simulink model "MODELODETURBINADERIO2017aV2"  (R2017b)
settings: Solver=FixedStepAuto  StartTime=0.0  StopTime=500  FixedStep=50e-3  RelTol=1e-3
values from neighbouring files (symbols this model uses):
  a = 790.51    [MODELOHIDRO.m]    (also in MODELOHIDROV2.m; MODELOHIDROV3.m)
  A = pi()*((D/2)^2)    [MODELOHIDRO.m]    (also in MODELOHIDROV10.m; MODELOHIDROV2.m; MODELOHIDROV3.m; MODELOHIDROV4.m)
  B = 0    [MODELOHIDRO.m]    (also in MODELOHIDROV10.m; MODELOHIDROV2.m; MODELOHIDROV3.m; MODELOHIDROV4.m)
  b = 6900.50    (= 6900.5)    [MODELOHIDRO.m]    (also in MODELOHIDROV2.m; MODELOHIDROV3.m)
  beta = 0    [MODELOHIDRO.m]    (also in MODELOHIDROV10.m; MODELOHIDROV2.m; MODELOHIDROV3.m; MODELOHIDROV4.m)
  Bi = 0.2287    [MODELOHIDRO.m]    (also in MODELOHIDROV10.m = 0.1; MODELOHIDROV2.m; MODELOHIDROV3.m; MODELOHIDROV4.m = 0.005)
  c = 23794    [MODELOHIDRO.m]    (also in MODELOHIDROV2.m; MODELOHIDROV3.m)
  d = 39268    [MODELOHIDRO.m]    (also in MODELOHIDROV2.m; MODELOHIDROV3.m)
  den = 1000    [MODELOHIDRO.m]    (also in MODELOHIDROV10.m; MODELOHIDROV2.m; MODELOHIDROV3.m; MODELOHIDROV4.m)
  e = 31863    [MODELOHIDRO.m]    (also in MODELOHIDROV2.m; MODELOHIDROV3.m)
  f = 10049    [MODELOHIDRO.m]    (also in MODELOHIDROV2.m; MODELOHIDROV3.m)
  J = 16.1919e-4    (= 0.00161919)    [MODELOHIDROV10.m]    (also in MODELOHIDROV2.m = 100; MODELOHIDROV3.m = 10; MODELOHIDROV4.m; MODELOHIDROV7.m)
  Ji = 1    [MODELOHIDRO.m]    (also in MODELOHIDROV10.m = 1.72; MODELOHIDROV2.m; MODELOHIDROV3.m; MODELOHIDROV4.m = 0.0465)
  k = 1    [MODELOHIDRO.m]    (also in MODELOHIDROV2.m; MODELOHIDROV3.m)
  Kb = 1.8    [MODELOHIDRO.m]    (also in MODELOHIDROV10.m = 6.2; MODELOHIDROV2.m; MODELOHIDROV3.m; MODELOHIDROV4.m = 0.027)
  Kp = 0.4    [MODELOHIDRO.m]    (also in MODELOHIDROV10.m = 5.6627; MODELOHIDROV2.m; MODELOHIDROV3.m; MODELOHIDROV4.m = 0.027)
  L_d = 38e-3    (= 0.038)    [MODELOHIDROV2.m]    (also in MODELOHIDROV3.m; MODELOHIDROV4.m; MODELOHIDROV7.m)
  L_q = 9.03e-3    (= 0.00903)    [MODELOHIDROV2.m]    (also in MODELOHIDROV3.m; MODELOHIDROV4.m; MODELOHIDROV7.m)
  Lambda = 0.48    [MODELOHIDROV2.m]    (also in MODELOHIDROV3.m; MODELOHIDROV4.m; MODELOHIDROV7.m)
  m = 5    [MODELOHIDRO.m]    (also in MODELOHIDROV2.m; MODELOHIDROV3.m)
  r = D/2    (= 0.5)    [MODELOHIDRO.m]    (also in MODELOHIDROV10.m; MODELOHIDROV2.m; MODELOHIDROV3.m; MODELOHIDROV4.m)
  Ri = 0.6    [MODELOHIDRO.m]    (also in MODELOHIDROV10.m = 0.973; MODELOHIDROV2.m; MODELOHIDROV3.m; MODELOHIDROV4.m = 1)
  Rs = 1.649    [MODELOHIDROV2.m]    (also in MODELOHIDROV3.m; MODELOHIDROV4.m; MODELOHIDROV7.m)
  T_d = 0    [MODELOHIDRO.m]    (also in MODELOHIDROV10.m; MODELOHIDROV2.m; MODELOHIDROV3.m; MODELOHIDROV4.m)
  z = 2    [MODELOHIDRO.m]    (also in MODELOHIDROV2.m; MODELOHIDROV3.m)
undefined symbols (not defined in the file or in its folder): sigbuilder_block
libraries: simulink x1
settings Model: Creator=zni.uao  LastModifiedBy=Hp 14
settings CodeAppCC: StateflowObjectComments=on
settings SimscapeCC: SimscapeNormalizeSystem=off

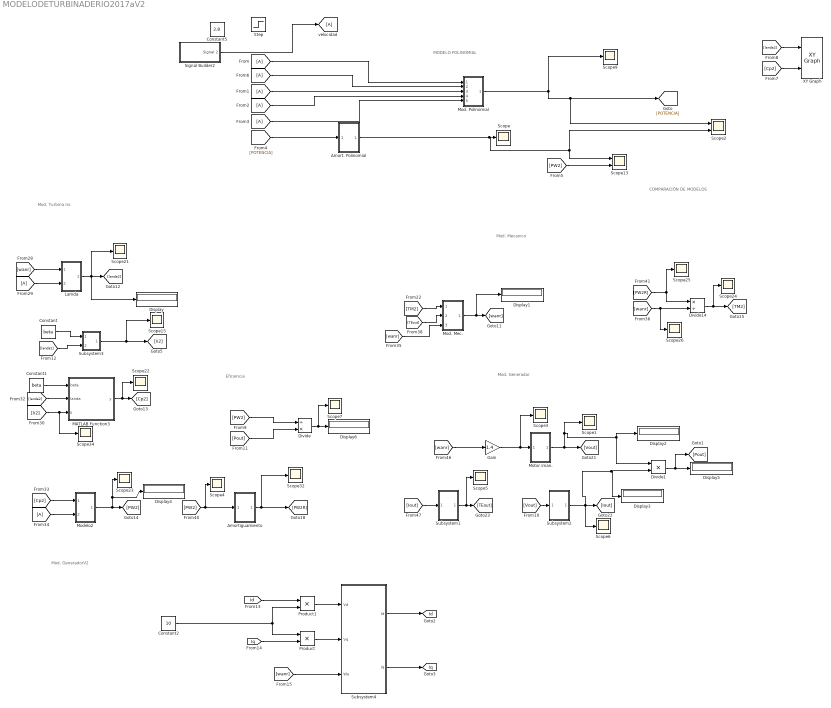
== system MODELODETURBINADERIO2017aV2 ==
  note: Mod. Generador
  note: MODELO POLINOMIAL
  note: COMPARACIÓN DE MODELOS
  note: Mod. Turbina rio
  note: Mod. Mecanico
  note: Mod. GeneradorV2
  note: Eficiencia
  Amort. Polinomial : Subsystem
  Amortiguamiento : Subsystem
  Constant : Constant  Value=beta
  Constant1 : Constant  Value=beta
  Constant2 : Constant  Value=10
  Constant5 : Constant  Value=2.8
  Display{,1..6} (7 alike) : Display
  Divide : Product  Inputs=/*
  Divide1 : Product  Inputs=**
  Divide14 : Product  Inputs=*/
  Gain : Gain  Gain=1.4
  Lamda : Subsystem
  MATLAB Function3 : MATLAB Function  TreatAsAtomicUnit=on
  Mod. Mec. : Subsystem
  Mod. Polinomial : Subsystem
  Modelo2 : Subsystem
  Motor iman. : Subsystem
  Product : Product
  Product1 : Product
  Scope{,1,3..7,9,15,21..26,32,34} (17 alike) : Scope
  Scope13 : Scope  NumInputPorts=2
  Scope2 : Scope  NumInputPorts=2
  Signal Builder2 : Subsystem  Tag=STV Subsys  LoadFcn=sigbuilder_block('load');  StartFcn=sigbuilder_block('start');  StopFcn=sigbuilder_block('stop');  ClipboardFcn=sigbuilder_block('clipboard');  mask(Sigbuilder block){tuvar=[0:10]}
      mask help: Simulink:masks:SigbuilderBlock_MD
      mask init:
      | if ~strcmp(get_param(bdroot(gcbh),'SimulationStatus'),'stopped') tuvar = sigbuilder_block('maskInit'); end
      settings: CopyFcn=sigbuilder_block('copy');  DeleteFcn=sigbuilder_block('delete');  ModelCloseFcn=sigbuilder_block('modelClose');  PreSaveFcn=sigbuilder_block('preSave');  PauseFcn=sigbuilder_block('pause');  ContinueFcn=sigbuilder_block('continue');  NameChangeFcn=sigbuilder_block('namechange');  OpenFcn=sigbuilder_block('open',[197.25 66 550.5 359.25 ]);  CloseFcn=sigbuilder_block('close');
      mask Display: plot(0, 0, 100, 100,[2, 2, 32, 32, 2], [68, 8, 8, 68, 68],[32, 2], [38, 38], [32, 19, 2],[53, 60, 44], [32, 17, 17, 2],[16, 16, 31, 31]);txt = getActiveGroup(gcbh);text(2, 100, txt,'verticalAlignment', 'top');
  Step : Step  Time=10  Before=2.5  After=2.888  SampleTime=0
  Subsystem1 : Subsystem
  Subsystem2 : Subsystem
  Subsystem3 : Subsystem
  Subsystem4 : Subsystem
  XY Graph : simulink/Sinks/XY Graph  xmin=1  xmax=20  ymin=0  ymax=0.56  st=0.1
  tag scope: Id=global, Iq=global
  wires:
  [landa2] -> XY Graph/1
  MATLAB Function3/1(y) -> [Cp2], Scope22/1
  Constant1/1 -> MATLAB Function3/1(beta)
  [landa2] -> MATLAB Function3/2(landa)
  [Ii2] -> Scope34/1, MATLAB Function3/3(Ii)
  Divide14/1 -> [TM2], Scope24/1
  [wanr] -> Scope26/1, Divide14/2
  [PW2R] -> Scope25/1, Divide14/1
  [PW2] -> Amortiguamiento/1(In1), Scope4/1
  Modelo2/1(Out1) -> Display4/1, Scope23/1, [PW2]
  [Cp2] -> Modelo2/1(In1)
  [A] -> Modelo2/2(In2)
  Lamda/1(Out1) -> Display/1, [landa2], Scope21/1
  [wanr] -> Lamda/1(In1)
  [A] -> Lamda/2(In2)
  [TM2] -> Mod. Mec./1(In1)
  [TEout] -> Mod. Mec./2(In2)
  Mod. Mec./1(Out1) -> Display1/1, [wanr]
  [Cp2] -> XY Graph/2
  Mod. Polinomial/1(Out1) -> Scope2/1, [POTENCIA], Scope9/1
  [A] -> Mod. Polinomial/1(In1)
  [A] -> Mod. Polinomial/2(In2)
  [A] -> Mod. Polinomial/3(In3)
  [A] -> Mod. Polinomial/4(In4)
  [A] -> Mod. Polinomial/5(In5)
  [wanr] -> Gain/1
  Motor iman./1(Out1) -> Divide1/1, Display2/1, Scope1/1, [Vout]
  Amortiguamiento/1(Out1) -> Scope32/1, [PW2R]
  Subsystem1/1(Out1) -> Scope5/1, [TEout]
  [Iout] -> Subsystem1/1(In1)
  Subsystem2/1(Out1) -> Divide1/2, Display3/1, Scope6/1, [Iout]
  [Vout] -> Subsystem2/1(In1)
  Subsystem3/1(Out1) -> Scope15/1, [Ii2]
  Constant/1 -> Subsystem3/1(In1)
  [landa2] -> Subsystem3/2(In2)
  [wanr] -> Mod. Mec./3(In3)
  Divide1/1 -> [Pout], Display5/1
  Amort. Polinomial/1(Out1) -> Scope2/2, Scope13/1, Scope/1
  [POTENCIA] -> Amort. Polinomial/1(In1)
  [PW2] -> Scope13/2
  Gain/1 -> Scope3/1, Motor iman./1(In1)
  [PW2] -> Divide/1
  [Pout] -> Divide/2
  Divide/1 -> Scope7/1, Display6/1
  Signal Builder2/1(Signal 2) -> [A]
  Subsystem4/1(Id) -> [Id]
  [Id] -> Product1/1
  [Iq] -> Product/2
  Constant2/1 -> Product/1, Product1/2
  Product/1 -> Subsystem4/2(Vq)
  Product1/1 -> Subsystem4/1(Vd)
  Subsystem4/2(Iq) -> [Iq]
  [wanr] -> Subsystem4/3(We)

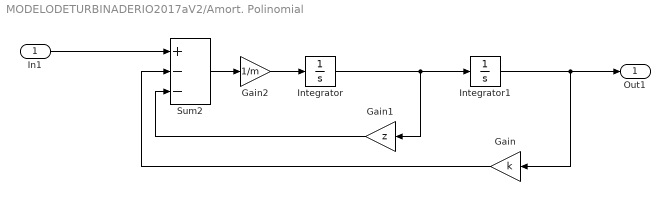
== system MODELODETURBINADERIO2017aV2/Amort. Polinomial ==
  In1 : Inport
  Gain : Gain  Gain=k
  Gain1 : Gain  Gain=z
  Gain2 : Gain  Gain=1/m
  Integrator : Integrator
  Integrator1 : Integrator
  Sum2 : Sum  Inputs=+--
  Out1 : Outport
  wires:
  Gain1/1 -> Sum2/3
  Sum2/1 -> Gain2/1
  Gain2/1 -> Integrator/1
  In1/1 -> Sum2/1
  Integrator/1 -> Gain1/1, Integrator1/1
  Gain/1 -> Sum2/2
  Integrator1/1 -> Out1/1, Gain/1

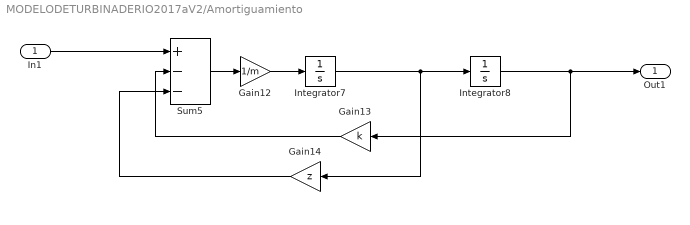
== system MODELODETURBINADERIO2017aV2/Amortiguamiento ==
  In1 : Inport
  Gain12 : Gain  Gain=1/m
  Gain13 : Gain  Gain=k
  Gain14 : Gain  Gain=z
  Integrator7 : Integrator
  Integrator8 : Integrator
  Sum5 : Sum  Inputs=+--
  Out1 : Outport
  wires:
  Gain13/1 -> Sum5/2
  Integrator8/1 -> Out1/1, Gain13/1
  Integrator7/1 -> Gain14/1, Integrator8/1
  Sum5/1 -> Gain12/1
  Gain12/1 -> Integrator7/1
  Gain14/1 -> Sum5/3
  In1/1 -> Sum5/1

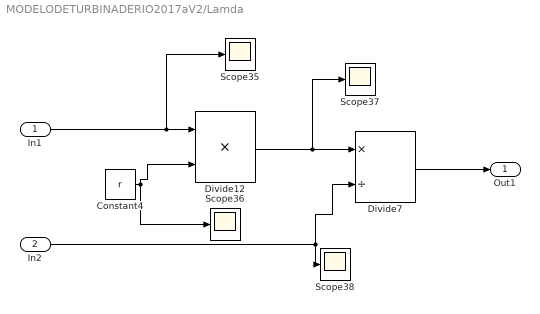
== system MODELODETURBINADERIO2017aV2/Lamda ==
  In1 : Inport
  In2 : Inport  Port=2
  Constant4 : Constant  Value=r
  Divide12 : Product  Inputs=**
  Divide7 : Product  Inputs=*/
  Scope{35..38} (4 alike) : Scope
  Out1 : Outport
  wires:
  Divide7/1 -> Out1/1
  Constant4/1 -> Divide12/2, Scope36/1
  In2/1 -> Divide7/2, Scope38/1
  Divide12/1 -> Scope37/1, Divide7/1
  In1/1 -> Scope35/1, Divide12/1

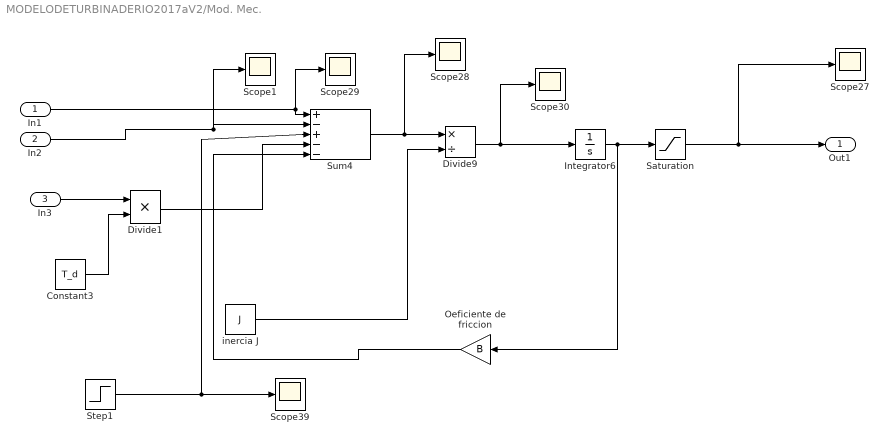
== system MODELODETURBINADERIO2017aV2/Mod. Mec. ==
  In1 : Inport
  In2 : Inport  Port=2
  In3 : Inport  Port=3
  Constant3 : Constant  Value=T_d
  Divide1 : Product  Inputs=**
  Divide9 : Product  Inputs=*/
  Integrator6 : Integrator  InitialCondition=10
  Oeficiente de friccion : Gain  Gain=B
  Saturation : Saturate  UpperLimit=44.5  LowerLimit=0
  Scope{1,27..30,39} (6 alike) : Scope
  Step1 : Step  Time=3  Before=5  After=0  SampleTime=0
  Sum4 : Sum  Inputs=|+-+--
  inercia J : Constant  Value=J
  Out1 : Outport
  wires:
  Oeficiente de friccion/1 -> Sum4/5
  In2/1 -> Scope1/1, Sum4/2
  inercia J/1 -> Divide9/2
  Divide9/1 -> Scope30/1, Integrator6/1
  Sum4/1 -> Scope28/1, Divide9/1
  Integrator6/1 -> Saturation/1, Oeficiente de friccion/1
  In1/1 -> Scope29/1, Sum4/1
  Step1/1 -> Scope39/1, Sum4/3
  Constant3/1 -> Divide1/2
  In3/1 -> Divide1/1
  Divide1/1 -> Sum4/4
  Saturation/1 -> Scope27/1, Out1/1

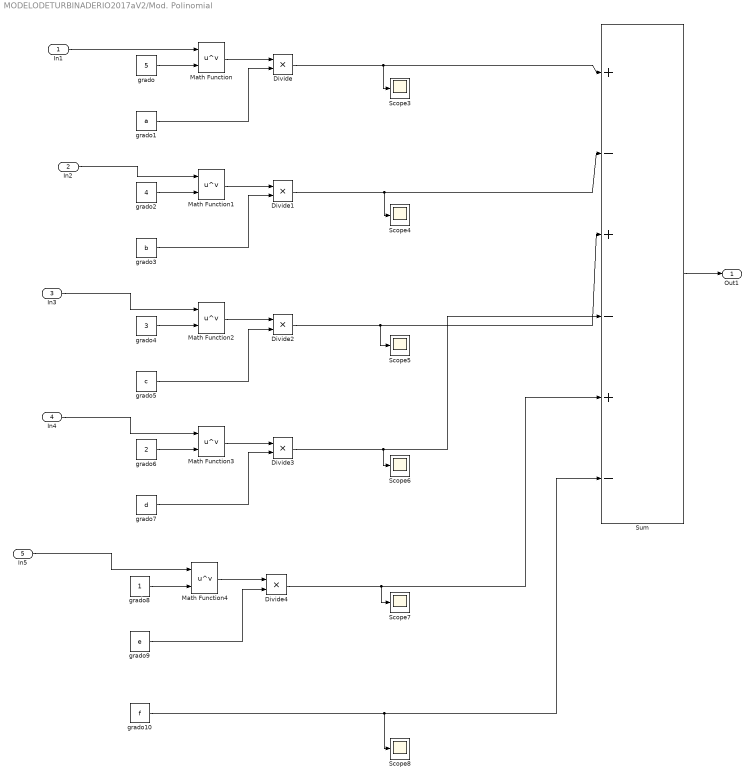
== system MODELODETURBINADERIO2017aV2/Mod. Polinomial ==
  In1 : Inport
  In2 : Inport  Port=2
  In3 : Inport  Port=3
  In4 : Inport  Port=4
  In5 : Inport  Port=5
  Divide{,1..4} (5 alike) : Product  Inputs=**
  Math Function{,1..4} (5 alike) : Math  Operator=pow  SaturateOnIntegerOverflow=on
  Scope{3..8} (6 alike) : Scope
  Sum : Sum  Inputs=|+-+-+-
  grado : Constant  Value=5
  grado1 : Constant  Value=a
  grado10 : Constant  Value=f
  grado2 : Constant  Value=4
  grado3 : Constant  Value=b
  grado4 : Constant  Value=3
  grado5 : Constant  Value=c
  grado6 : Constant  Value=2
  grado7 : Constant  Value=d
  grado8 : Constant
  grado9 : Constant  Value=e
  Out1 : Outport
  wires:
  In3/1 -> Math Function2/1
  Sum/1 -> Out1/1
  grado/1 -> Math Function/2
  grado9/1 -> Divide4/2
  grado3/1 -> Divide1/2
  In1/1 -> Math Function/1
  Math Function/1 -> Divide/1
  Divide2/1 -> Sum/3, Scope5/1
  grado2/1 -> Math Function1/2
  grado7/1 -> Divide3/2
  Divide3/1 -> Scope6/1, Sum/4
  grado10/1 -> Scope8/1, Sum/6
  Math Function3/1 -> Divide3/1
  Divide4/1 -> Scope7/1, Sum/5
  In2/1 -> Math Function1/1
  grado4/1 -> Math Function2/2
  Math Function1/1 -> Divide1/1
  grado1/1 -> Divide/2
  grado5/1 -> Divide2/2
  Math Function4/1 -> Divide4/1
  Divide/1 -> Scope3/1, Sum/1
  Math Function2/1 -> Divide2/1
  Divide1/1 -> Scope4/1, Sum/2
  In5/1 -> Math Function4/1
  In4/1 -> Math Function3/1
  grado6/1 -> Math Function3/2
  grado8/1 -> Math Function4/2

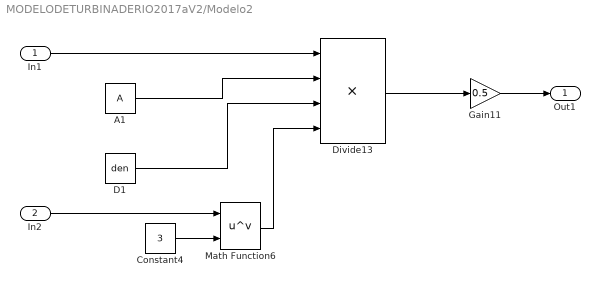
== system MODELODETURBINADERIO2017aV2/Modelo2 ==
  In1 : Inport
  In2 : Inport  Port=2
  A1 : Constant  Value=A
  Constant4 : Constant  Value=3
  D1 : Constant  Value=den
  Divide13 : Product  Inputs=****  SaturateOnIntegerOverflow=on  RndMeth=Zero
  Gain11 : Gain  Gain=0.5
  Math Function6 : Math  Operator=pow  SaturateOnIntegerOverflow=on
  Out1 : Outport
  wires:
  Constant4/1 -> Math Function6/2
  Divide13/1 -> Gain11/1
  D1/1 -> Divide13/3
  In1/1 -> Divide13/1
  Gain11/1 -> Out1/1
  A1/1 -> Divide13/2
  In2/1 -> Math Function6/1
  Math Function6/1 -> Divide13/4

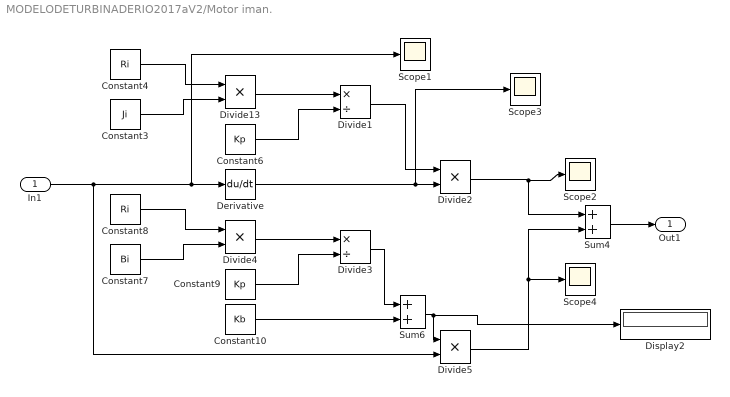
== system MODELODETURBINADERIO2017aV2/Motor iman. ==
  In1 : Inport
  Constant10 : Constant  Value=Kb
  Constant3 : Constant  Value=Ji
  Constant4 : Constant  Value=Ri
  Constant6 : Constant  Value=Kp
  Constant7 : Constant  Value=Bi
  Constant8 : Constant  Value=Ri
  Constant9 : Constant  Value=Kp
  Derivative : Derivative
  Display2 : Display
  Divide1 : Product  Inputs=*/  SaturateOnIntegerOverflow=on  RndMeth=Zero
  Divide{2,4..5,13} (4 alike) : Product  Inputs=**  SaturateOnIntegerOverflow=on  RndMeth=Zero
  Divide3 : Product  Inputs=*/  SaturateOnIntegerOverflow=on  RndMeth=Zero
  Scope{1..4} (4 alike) : Scope
  Sum4 : Sum
  Sum6 : Sum
  Out1 : Outport
  wires:
  Constant10/1 -> Sum6/2
  Divide2/1 -> Scope2/1, Sum4/1
  In1/1 -> Divide5/2, Scope1/1, Derivative/1
  Divide3/1 -> Sum6/1
  Divide13/1 -> Divide1/1
  Constant6/1 -> Divide1/2
  Constant4/1 -> Divide13/1
  Sum6/1 -> Display2/1, Divide5/1
  Divide1/1 -> Divide2/1
  Constant3/1 -> Divide13/2
  Constant9/1 -> Divide3/2
  Divide4/1 -> Divide3/1
  Constant7/1 -> Divide4/2
  Constant8/1 -> Divide4/1
  Derivative/1 -> Scope3/1, Divide2/2
  Sum4/1 -> Out1/1
  Divide5/1 -> Scope4/1, Sum4/2

== system MODELODETURBINADERIO2017aV2/Signal Builder2 ==
  Demux : Demux  Tag=STV Demux  Outputs=1
  FromWs : FromWorkspace  Tag=STV FromWs  VariableName=tuvar  SampleTime=0
      SigBuilderData=|
      | common.afterFinalStr = 'Extrapolate'
      | common.sampleTime = 0
      | dataSet.timeRange = [0 10]
      | dataSet.name = 'Group 1'
      | sbobj.Groups.Name = 'Group 1'
      | sbobj.Groups.Signals.Name = 'Signal 2'
      | sbobj.Groups.Signals.XData = [0 3 3 5 5 10]
      | sbobj.Groups.Signals.YData = [2 2 2.5 2.5 2.8 2.8]
  Signal 2 : Outport  Tag=STV Outport
  wires:
  FromWs/1 -> Demux/1
  Demux/1 -> Signal 2/1

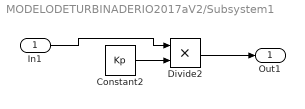
== system MODELODETURBINADERIO2017aV2/Subsystem1 ==
  In1 : Inport
  Constant2 : Constant  Value=Kp
  Divide2 : Product  Inputs=**
  Out1 : Outport
  wires:
  In1/1 -> Divide2/1
  Constant2/1 -> Divide2/2
  Divide2/1 -> Out1/1

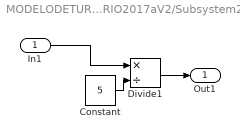
== system MODELODETURBINADERIO2017aV2/Subsystem2 ==
  In1 : Inport
  Constant : Constant  Value=5
  Divide1 : Product  Inputs=*/
  Out1 : Outport
  wires:
  Divide1/1 -> Out1/1
  Constant/1 -> Divide1/2
  In1/1 -> Divide1/1

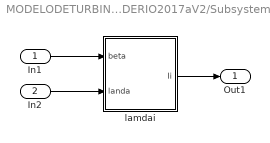
== system MODELODETURBINADERIO2017aV2/Subsystem3 ==
  In1 : Inport
  In2 : Inport  Port=2
  lamdai : MATLAB Function  TreatAsAtomicUnit=on
  Out1 : Outport
  wires:
  lamdai/1(Ii) -> Out1/1
  In2/1 -> lamdai/2(landa)
  In1/1 -> lamdai/1(beta)

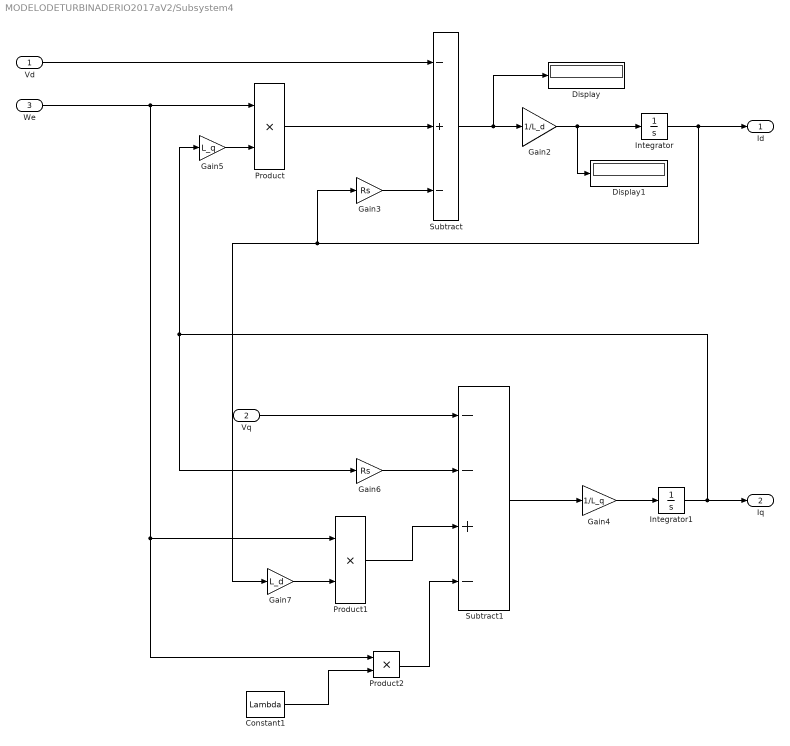
== system MODELODETURBINADERIO2017aV2/Subsystem4 ==
  Vd : Inport
  Vq : Inport  Port=2
  We : Inport  Port=3
  Constant1 : Constant  Value=Lambda
  Display : Display
  Display1 : Display
  Gain2 : Gain  Gain=1/L_d
  Gain3 : Gain  Gain=Rs
  Gain4 : Gain  Gain=1/L_q
  Gain5 : Gain  Gain=L_q
  Gain6 : Gain  Gain=Rs
  Gain7 : Gain  Gain=L_d
  Integrator : Integrator
  Integrator1 : Integrator
  Product : Product
  Product1 : Product
  Product2 : Product
  Subtract : Sum  Inputs=-+-
  Subtract1 : Sum  Inputs=--+-
  Id : Outport
  Iq : Outport  Port=2
  wires:
  Integrator1/1 -> Gain6/1, Gain5/1, Iq/1
  We/1 -> Product/1, Product2/1, Product1/1
  Product1/1 -> Subtract1/3
  Gain7/1 -> Product1/2
  Product/1 -> Subtract/2
  Integrator/1 -> Id/1, Gain7/1, Gain3/1
  Gain4/1 -> Integrator1/1
  Gain2/1 -> Display1/1, Integrator/1
  Gain5/1 -> Product/2
  Subtract/1 -> Display/1, Gain2/1
  Subtract1/1 -> Gain4/1
  Vq/1 -> Subtract1/1
  Gain6/1 -> Subtract1/2
  Vd/1 -> Subtract/1
  Constant1/1 -> Product2/2
  Product2/1 -> Subtract1/4
  Gain3/1 -> Subtract/3

== matlab function MODELODETURBINADERIO2017aV2/MATLAB Function3 ==
  data: beta input; y output; landa input; Ii input
function y = fcn(beta, landa,Ii)
w=0.5176; 
w1=116/Ii;
 w2=0.4*beta;
 w3=exp(-21/Ii);
 
 cp=w*(w1-w2-5)*w3+0.0068*landa;
 
 
 
 
 
y=cp;

== matlab function MODELODETURBINADERIO2017aV2/Subsystem3/lamdai ==
  data: beta input; Ii output; landa input
function Ii = fcn(beta,landa)


Iii=(1/((landa+(0.08*beta))))-((0.035)/((beta^3)+1));
Ii=1/Iii;
